simulink model "Elevacion3"  (R2025b)
settings: Solver=VariableStepAuto  StartTime=0.0  StopTime=30.0  RelTol=1e-3
libraries: simulink x1
settings Model: Creator=alfon  LastModifiedBy=alfon

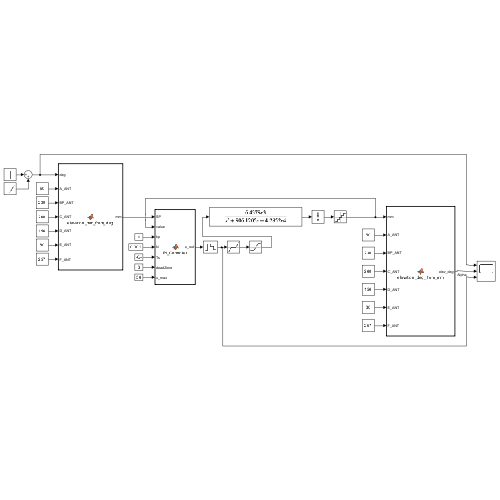
[thumbnail: Simulink's stored preview of the top-level diagram]
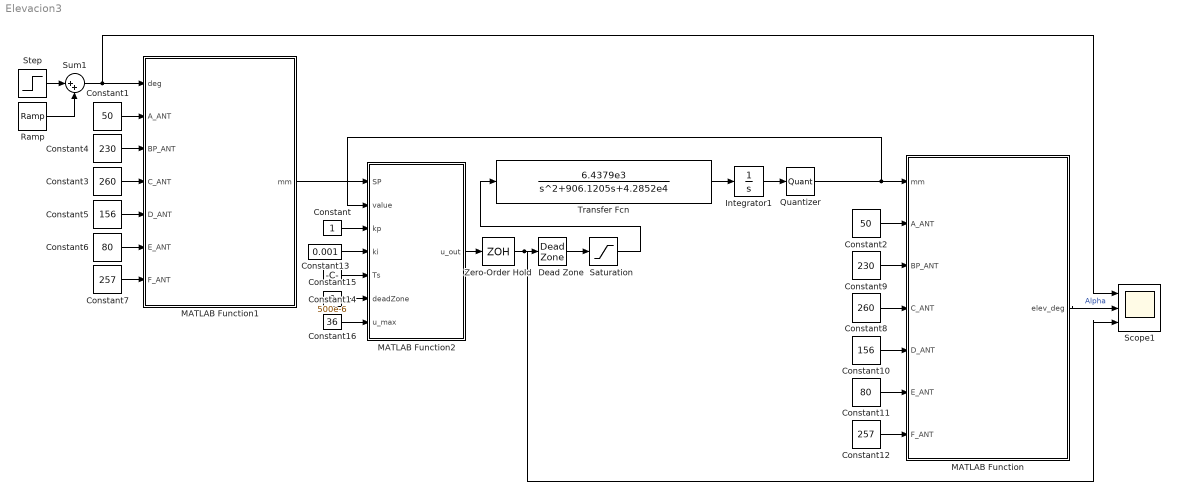
== system Elevacion3 ==
  Constant : Constant
  Constant1 : Constant  Value=50
  Constant10 : Constant  Value=156
  Constant11 : Constant  Value=80
  Constant12 : Constant  Value=257
  Constant13 : Constant  Value=0.001
  Constant14 : Constant  Value=500e-6
  Constant15 : Constant  Value=3
  Constant16 : Constant  Value=36
  Constant2 : Constant  Value=50
  Constant3 : Constant  Value=260
  Constant4 : Constant  Value=230
  Constant5 : Constant  Value=156
  Constant6 : Constant  Value=80
  Constant7 : Constant  Value=257
  Constant8 : Constant  Value=260
  Constant9 : Constant  Value=230
  Dead Zone : DeadZone  LowerValue=-3  UpperValue=3
  Integrator1 : Integrator
  MATLAB Function : MATLAB Function  TreatAsAtomicUnit=on
  MATLAB Function1 : MATLAB Function  TreatAsAtomicUnit=on
  MATLAB Function2 : MATLAB Function  TreatAsAtomicUnit=on  SystemSampleTime=500e-6
  Quantizer : Quantizer  QuantizationInterval=1.6
  Ramp : simulink/Sources/Ramp  slope=-0.05  start=0  InitialOutput=0
  Saturation : Saturate  UpperLimit=36  LowerLimit=-36
  Scope1 : Scope  NumInputPorts=3
      settings: ActiveDisplayYMinimum=-6.1785685922162061  ActiveDisplayYMaximum=100.84612358117622
  Step : Step  Time=0  After=75  SampleTime=0
  Sum1 : Sum  Inputs=|++
  Transfer Fcn : TransferFcn  Numerator=[6.4379e3]  Denominator=[1,906.1205,4.2852e4]
  Zero-Order Hold : ZeroOrderHold  SampleTime=-1
  wires:
  Constant3/1 -> MATLAB Function1/4(C_ANT)
  Constant4/1 -> MATLAB Function1/3(BP_ANT)
  Constant5/1 -> MATLAB Function1/5(D_ANT)
  Constant1/1 -> MATLAB Function1/2(A_ANT)
  Step/1 -> Sum1/1
  Constant11/1 -> MATLAB Function/6(E_ANT)
  Constant7/1 -> MATLAB Function1/7(F_ANT)
  Sum1/1 -> Scope1/1, MATLAB Function1/1(deg)
  Constant10/1 -> MATLAB Function/5(D_ANT)
  Transfer Fcn/1 -> Integrator1/1
  Constant6/1 -> MATLAB Function1/6(E_ANT)
  MATLAB Function/1(elev_deg) -> Scope1/2  "Alpha"
  Constant9/1 -> MATLAB Function/3(BP_ANT)
  Constant12/1 -> MATLAB Function/7(F_ANT)
  Dead Zone/1 -> Saturation/1
  Saturation/1 -> Transfer Fcn/1
  Constant2/1 -> MATLAB Function/2(A_ANT)
  Integrator1/1 -> Quantizer/1
  Ramp/1 -> Sum1/2
  Constant8/1 -> MATLAB Function/4(C_ANT)
  Constant15/1 -> MATLAB Function2/6(deadZone)
  Constant16/1 -> MATLAB Function2/7(u_max)
  Constant/1 -> MATLAB Function2/3(kp)
  MATLAB Function2/1(u_out) -> Zero-Order Hold/1
  Constant13/1 -> MATLAB Function2/4(ki)
  Constant14/1 -> MATLAB Function2/5(Ts)
  MATLAB Function1/1(mm) -> MATLAB Function2/1(SP)
  Zero-Order Hold/1 -> Dead Zone/1, Scope1/3
  Quantizer/1 -> MATLAB Function2/2(value), MATLAB Function/1(mm)

== matlab function Elevacion3/MATLAB Function1 ==
  data: deg input; mm output; A_ANT input; BP_ANT input; C_ANT input; D_ANT input; E_ANT input; F_ANT input
function mm = elevation_mm_from_deg(deg, A_ANT, BP_ANT, C_ANT, D_ANT, E_ANT, F_ANT)
A_CONST = 3*pi/2 - atan2(C_ANT, D_ANT) - atan2(F_ANT, E_ANT);

B_CONST = 2 * sqrt( (F_ANT^2 + E_ANT^2) * (D_ANT^2 + C_ANT^2) );

C_CONST = F_ANT^2 + E_ANT^2 + D_ANT^2 + C_ANT^2 - A_ANT^2;

DEG_TO_RAD = pi/180;

mm = sqrt(C_CONST - B_CONST * cos(A_CONST - DEG_TO_RAD * deg)) - BP_ANT;

end

== matlab function Elevacion3/MATLAB Function ==
  data: mm input; elev_deg output; A_ANT input; BP_ANT input; C_ANT input; D_ANT input; E_ANT input; F_ANT input
function elev_deg = elevation_deg_from_mm(mm, A_ANT, BP_ANT, C_ANT, D_ANT, E_ANT, F_ANT)

A_CONST = 3*pi/2 - atan2(C_ANT, D_ANT) - atan2(F_ANT, E_ANT);

B_CONST = 2 * sqrt((F_ANT^2 + E_ANT^2) * (D_ANT^2 + C_ANT^2));

C_CONST = F_ANT^2 + E_ANT^2 + D_ANT^2 + C_ANT^2 - A_ANT^2;

elev_deg = (A_CONST - acos((C_CONST - (BP_ANT + mm)^2) / B_CONST)) * 180/pi;
end

== matlab function Elevacion3/MATLAB Function2 ==
  data: SP input; u_out output; value input; kp input; ki input; Ts input; deadZone input; u_max input
function u_out = PI_Controller(SP, value, kp, ki, Ts, deadZone, u_max)

    persistent e1 u1 v_f

    if isempty(e1)
        e1 = 0;
        u1 = 0;
        v_f = 0;
    end

    % -------- Low-pass filter --------
    fc = 0.1;                           % Hz
    alpha = exp(-2*pi*fc*Ts);
    v_f = alpha*v_f + (1-alpha)*value;

    % -------- PI (Tustin incremental) --------
    a = kp + (ki*Ts)/2;
    b = -kp + (ki*Ts)/2;

    e0 = SP - v_f;
    u0 = u1 + a*e0 + b*e1;

    % -------- Dead-zone compensation --------
    if u0 > 0
        u_dz = u0 + deadZone;
    elseif u0 < 0
        u_dz = u0 - deadZone;
    else
        u_dz = 0;
    end
    
    
    % -------- Saturation --------
    u_sat = min(max(u_dz, -u_max), u_max);

    % -------- Anti-windup --------
    if abs(u_sat) <= u_max
        u1 = u0;
        e1 = e0;
    end

    u_out = u_sat;
end
